simulink model "Exp ed"  (R2016a)
settings: Solver=VariableStepAuto  StartTime=0.0  StopTime=1  RelTol=1e-3
settings Model: Creator=PAPUN  LastModifiedBy=PAPUN

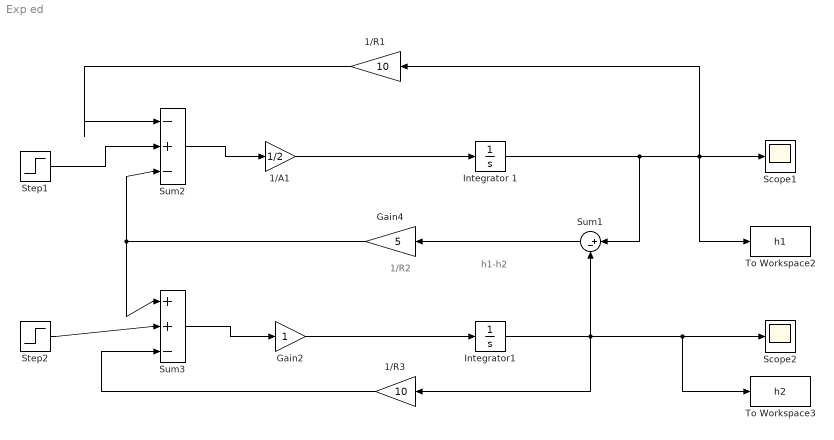
== system Exp ed ==
  note: 1/R2
  note: h1-h2
  1/A1 : Gain  Gain=1/2
  1/R1 : Gain  Gain=10
  1/R3 : Gain  Gain=10
  Gain2 : Gain
  Gain4 : Gain  Gain=5
  Integrator 1 : Integrator
  Integrator1 : Integrator
  Scope1 : Scope
  "Scope2 " : Scope
  Step1 : Step  SampleTime=0
  Step2 : Step  SampleTime=0
  Sum1 : Sum  Inputs=|+-
  Sum2 : Sum  Inputs=|-+-
  Sum3 : Sum  Inputs=|++-
  To Workspace2 : ToWorkspace  VariableName=h1  SampleTime=-1
      settings: Save2DSignal=2-D array (concatenate along first dimension)
  To Workspace3 : ToWorkspace  VariableName=h2  SampleTime=-1
      settings: Save2DSignal=2-D array (concatenate along first dimension)
  wires:
  1/A1/1 -> Integrator 1/1
  Gain2/1 -> Integrator1/1
  Step1/1 -> Sum2/2
  Step2/1 -> Sum3/2
  1/R1/1 -> Sum2/1
  Integrator 1/1 -> 1/R1/1, To Workspace2/1, Scope1/1, Sum1/1
  Integrator1/1 -> 1/R3/1, Sum1/2, To Workspace3/1, "Scope2 "/1
  Sum1/1 -> Gain4/1
  1/R3/1 -> Sum3/3
  Sum3/1 -> Gain2/1
  Sum2/1 -> 1/A1/1
  Gain4/1 -> Sum3/1, Sum2/3
